simulink model "Lab1_NomPlantModel_V2"  (R2019a)
settings: Solver=VariableStepAuto  StartTime=0.0  StopTime=100  RelTol=1e-3
libraries: cstblocks x1
settings Model: Creator=emma  LastModifiedBy=emma

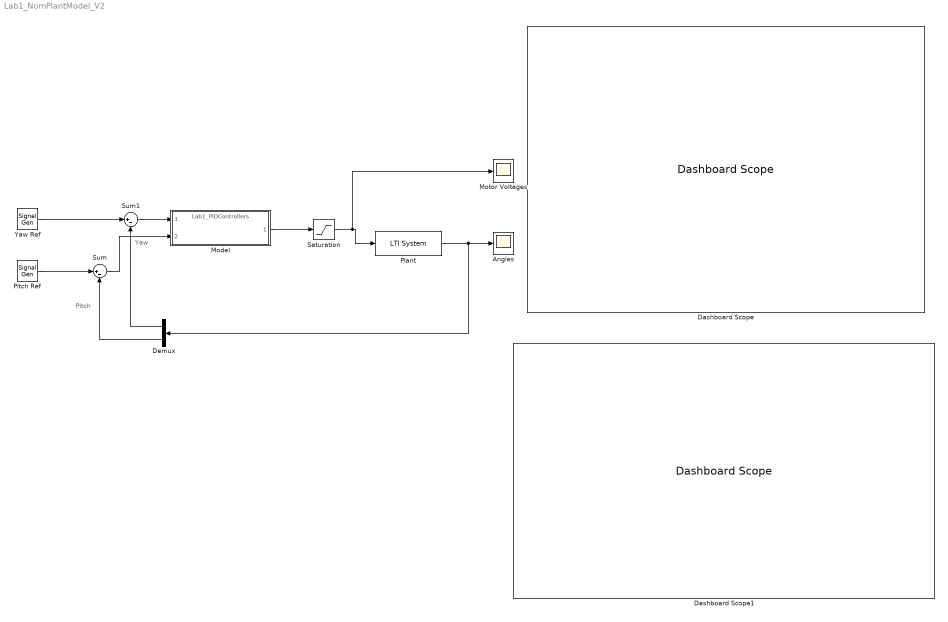
== system Lab1_NomPlantModel_V2 ==
  note: Yaw
  note: Pitch
  Angles : Scope
  Dashboard Scope : DashboardScope
  Dashboard Scope1 : DashboardScope
  Demux : Demux  Outputs=2
  Model : ModelReference  ModelNameDialog=Lab1_PIDControllers.slx  SimulationMode=Normal  ModelReferenceVersion=1.2
  Motor Voltages : Scope
  Pitch Ref : SignalGenerator  WaveForm=square  Amplitude=pi/6  Frequency=0.4  Units=rad/sec
  Plant : cstblocks/LTI System  sys=Gnom  IC=[]
  Saturation : Saturate  UpperLimit=+25  LowerLimit=-25
  Sum : Sum  Inputs=|+-
  Sum1 : Sum  Inputs=|+-
  Yaw Ref : SignalGenerator  WaveForm=square  Amplitude=pi/4  Frequency=0.5  Units=rad/sec
  wires:
  Yaw Ref/1 -> Sum1/1
  Plant/1 -> Demux/1, Angles/1
  Pitch Ref/1 -> Sum/1
  Demux/1 -> Sum1/2
  Demux/2 -> Sum/2
  Sum1/1 -> Model/1
  Sum/1 -> Model/2
  Model/1 -> Saturation/1
  Saturation/1 -> Motor Voltages/1, Plant/1
